simulink model "untitled1"  (R2020b)
settings: Solver=VariableStepAuto  StartTime=0.0  StopTime=10.0  RelTol=1e-3
libraries: mcl x2
settings Model: Creator=sai  LastModifiedBy=sai

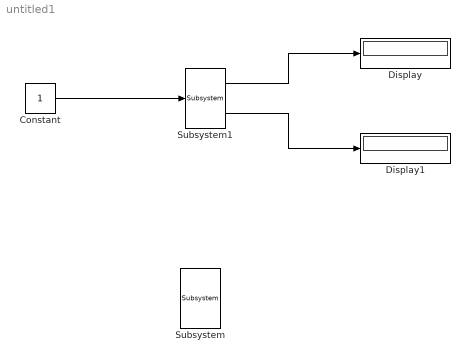
== system untitled1 ==
  Constant : Constant
  Display : Display
  Display1 : Display
  Subsystem : mcl/Subsystem  A=33  B=44
  Subsystem1 : mcl/Subsystem  A=33  B=44
  wires:
  Constant/1 -> Subsystem1/1
  Subsystem1/1 -> Display/1
  Subsystem1/2 -> Display1/1
